simulink model "L5E1"  (R2020b)
settings: Solver=VariableStepAuto  StartTime=0.0  StopTime=10.0  RelTol=1e-3
settings Model: Creator=Vedant Nath  LastModifiedBy=Vedant Nath

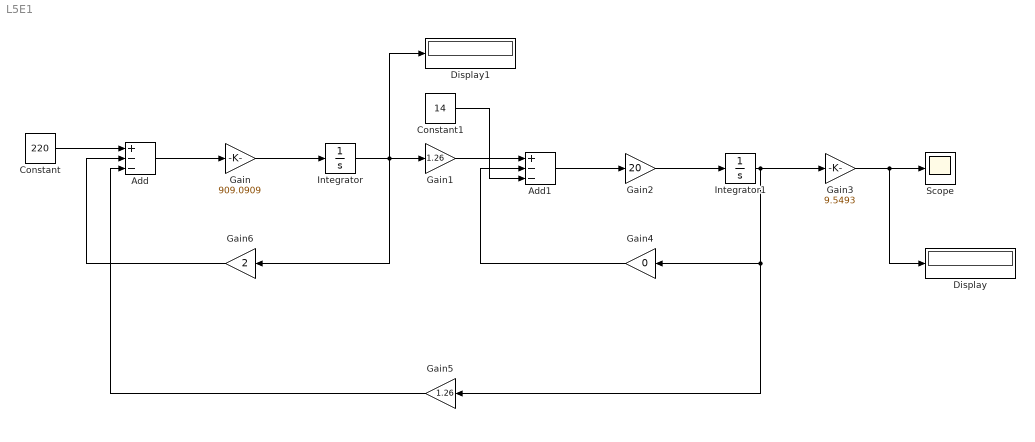
== system L5E1 ==
  Add : Sum  Inputs=+--
  Add1 : Sum  Inputs=+--
  Constant : Constant  Value=220
  Constant1 : Constant  Value=14
  Display : Display
  Display1 : Display
  Gain : Gain  Gain=909.0909
  Gain1 : Gain  Gain=1.26
  Gain2 : Gain  Gain=20
  Gain3 : Gain  Gain=9.5493
  Gain4 : Gain  Gain=0
  Gain5 : Gain  Gain=1.26
  Gain6 : Gain  Gain=2
  Integrator : Integrator
  Integrator1 : Integrator
  Scope : Scope
  wires:
  Constant/1 -> Add/1
  Add/1 -> Gain/1
  Gain/1 -> Integrator/1
  Integrator/1 -> Display1/1, Gain6/1, Gain1/1
  Gain1/1 -> Add1/1
  Gain2/1 -> Integrator1/1
  Add1/1 -> Gain2/1
  Integrator1/1 -> Gain5/1, Gain4/1, Gain3/1
  Gain4/1 -> Add1/2
  Gain3/1 -> Scope/1, Display/1
  Constant1/1 -> Add1/3
  Gain5/1 -> Add/3
  Gain6/1 -> Add/2
